simulink model "sbc_uja113x_mode_control_s32k148"  (Simulink 9.0)
settings: Solver=FixedStepDiscrete  StartTime=0.0  StopTime=10.0  FixedStep=0.1  RelTol=1e-3
InitFcn:
  | mbd_s32k_consistency_checks(bdroot(gcs));
undefined symbols (not defined in the file): bit, LQFP
libraries: mbd_s32k1xx_ec_toolbox x12, mbd_sbc_ec_toolbox x7, simulink x1
Description:
  | This model demonstrates how to handle operating modes of SBC.
  | 
  | Validation:
  | - A BLUE led is toggled at each time Watchdog resets
  | - Press SW3 to send SBC in Standby mode (RED led should be on)
  | - Press SW4 to send SBC in Normal mode (GREEN led should be on)
  | 
  | Note:
  | This application flashes the non-volatile memory MTPNV and configures the SBC in non-FNMC mode.
  | While the SBC is in non-FNMC mode, the device starts to pull the reset line.
  | It is recommended to clear the MTPNV memory, after this example.
  | 
  |  Erasing the MTPNV memory:
  |  - Connect J11-1 (CANH) to J13-2 (LIN1 VBAT)
  |  - Connect J11-2 (CANL) to J11-4 (GND)
  |  - Push and hold down the reset button SW5
  |  - Turn off and on  the 12V power supply
  |  - Release the reset button and remove the jumper wires
  | 
  | HW prerequisite:
  | - S32k148EVB
  | - One Power Adapter 12V
settings Model: Creator=nxf35375  LastModifiedBy=nxf35172
settings DataIOCC: ExternalInput=off  InitialState=off  SaveFormat=Dataset  SaveOutput=off  SignalLogging=off  SaveTime=off
settings OptimizationCC: DefaultParameterBehavior=Inlined  PassReuseOutputArgsAs=Individual arguments  LifeSpan=auto
settings DebuggingCC: UnderspecifiedInitializationDetection=Simplified  MergeDetectMultiDrivingBlocksExec=error  InheritedTsInSrcMsg=none  SingleTaskRateTransMsg=error  ParameterTunabilityLossMsg=error  UnconnectedInputMsg=error  UnconnectedOutputMsg=error  UnconnectedLineMsg=error  UnknownTsInhSupMsg=error  SFUnexpectedBacktrackingDiag=error  SFNoUnconditionalDefaultTransitionDiag=error  SFExecutionAtInitializationDiag=warning
settings HardwareCC: ProdLargestAtomicInteger=Long  ProdLargestAtomicFloat=Double  ProdIntDivRoundTo=Zero  ProdEndianess=LittleEndian  ProdHWDeviceType=ARM Compatible->ARM Cortex
settings ModelReferenceCC: PropagateSignalLabelsOutOfModel=on
settings SFSimCC: MATLABDynamicMemAlloc=off
settings RTWCC: SystemTargetFile=mbd_s32k.tlc  MakeCommand=mbd_s32k_make_rtw COPY_MDLREF_INCLUDES=0  TemplateMakefile=mbd_s32k.tmf  Description=Model Based Design Toolbox S32K14x Code Generation Target  GenerateReport=on  IncludeHyperlinkInReport=on  LaunchReport=on  GenerateTraceInfo=on  GenerateTraceReport=on  GenerateTraceReportSl=on  GenerateTraceReportSf=on  GenerateTraceReportEml=on
settings CodeAppCC: ForceParamTrailComments=on  IgnoreCustomStorageClasses=off  OperatorAnnotations=on  SimulinkDataObjDesc=on  SFDataObjDesc=on  InsertBlockDesc=on  StateflowObjectComments=off
settings STFCustomTargetCC: TargetLangStandard=C99 (ISO)  MultiwordLength=256  CombineOutputUpdateFcns=on  ERTCustomFileBanners=on  SupportContinuousTime=off  SupportNonInlinedSFcns=off  RemoveResetFunc=on  MATLABClassNameForMDSCustomization=Simulink.SoftwareTarget.ERTCustomization  GRTInterface=off  SystemTargetFile=mbd_s32k.tlc
settings ERTTargetCC: TargetLangStandard=C99 (ISO)  ParMdlRefBuildCompliant=off  CompOptLevelCompliant=off  ConcurrentExecutionCompliant=off  ModelStepFunctionPrototypeControlCompliant=off  CPPClassGenCompliant=off  UseToolchainInfoCompliant=off  InlinedParameterPlacement=NonHierarchical  ERTSrcFileBannerTemplate=mbd_ert_code_template.cgt  ERTHdrFileBannerTemplate=mbd_ert_code_template.cgt  ERTDataSrcFileTemplate=mbd_ert_code_template.cgt  ERTDataHdrFileTemplate=mbd_ert_code_template.cgt  ERTCustomFileTemplate=example_file_process.tlc
settings ConfigComp: CovMetricSettings=dwe  CovHtmlReporting=off  CovSaveCumulativeToWorkspaceVar=off  CovSaveSingleToWorkspaceVar=off  CovExternalEMLEnable=on

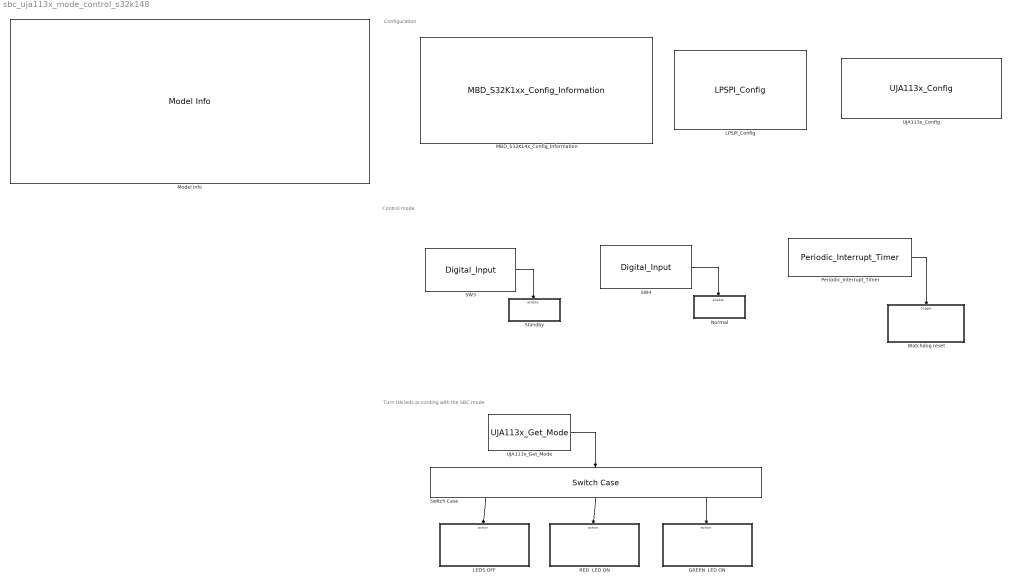
== system sbc_uja113x_mode_control_s32k148 ==
  note: Configuration
  note: Control mode
  note: Turn ON leds according with the SBC mode
  GREEN  LED ON : Subsystem  TreatAsAtomicUnit=on
  LEDS OFF : Subsystem  TreatAsAtomicUnit=on
  "LPSPI_Config " : mbd_s32k1xx_ec_toolbox/Communication Blocks/SPI Blocks/LPSPI_Config   Priority=1  InstanceNumber=1  Role=Master  BaudRate=4000000  ShowAdvanced=on  sin=PTA29: [LPSPI1_SIN | LPSPI Serial Data Input]  sout=PTA27: [LPSPI1_SOUT | LPSPI Serial Data Output]  sck=PTA28: [LPSPI1_SCK | LPSPI Serial Clock I/O]  pcs0=PTA26: [LPSPI1_PCS0 | Peripheral Chip Select 0]  pcs1=None  pcs2=None  pcs3=None  CPHA=1  CPOL=0  BitOrder=MSB first  TransferSize=8  WhichPCS=0  PCSPol=ActiveLow  ContinuousTransfer=on
  MBD_S32K14x_Config_Information : mbd_s32k1xx_ec_toolbox/MBD_S32K1xx_Config_Information  mbdt_ver=0  disp_str=|  config_params=[]  mcu_target_name=S32K148  mcu_target_package=144-LQFP  mcu_target_sram_size=192KB  mcu_system_clock_freq=80  mcu_xtal_freq=External 8  mcu_steptick_timer=LPIT Channel 0  mcu_steptick_prio=15  ds_import_enable=on  target_compiler=GCC  target_memory=FLASH  gcc_target_compile_opts=-mcpu=cortex-m4 -mthumb -mfloat-abi=hard -mfpu=fpv4-sp-d16 -O1 -g -gstrict-dwarf  gcc_target_assemble_opts=-mcpu=cortex-m4 -mthumb -mfloat-abi=hard -mfpu=fpv4-sp-d16 -g  gcc_target_link_opts=-mcpu=cortex-m4 -mthumb -mfloat-abi=hard -mfpu=fpv4-sp-d16  gcc_target_default_lcf=on  gcc_target_user_lcf=S32K148_192_flash.ld  ghs_target_compile_opts=-cpu=cortexm4f -thumb -DARM_MATH_CM4 -fpu=vfpv4_d16 -fsingle -Ogeneral -Wundef -Wimplicit-int -Wshadow -Wtrigraphs --no_commons --gnu_asm -gnu99 -gdwarf-2 -G  ghs_target_assemble_opts=-cpu=cortexm4f -fpu=vfpv4_d16  ghs_target_link_opts=-cpu=cortexm4f -thumb -fpu=vfpv4_d16  ghs_target_default_lcf=off  ghs_target_user_lcf=S32K148_192_flash.ld  iar_target_compile_opts=--cpu=Cortex-M4F --thumb --fpu=VFPv4_sp -Ol -e --debug --dlib_config normal  iar_target_assemble_opts=--cpu Cortex-M4F --thumb --fpu VFPv4_sp  iar_target_link_opts=--no_exceptions --vfe --inline  iar_target_default_lcf=off  iar_target_user_lcf=S32K148_192_flash.icf  pil_download_enable=off  rbl_download_enable=on  rbl_start_delay=5000000  rbl_download_interface=OpenSDA  rbl_restart_request=off  rbl_com_port=Custom  rbl_com_port_custom=COM1  pil_download_rate=57600  pil_opensda_drive=Custom  pil_opensda_drive_custom=D  pil_uart_instance=0  pil_uart_rx=PTA2: [LPUART0_RX | Receive]  pil_uart_tx=PTA3: [LPUART0_TX | Transmit]  FTM_PWM_PcrCheckEnDis=on  FTM_Input_Edge_Inputs_PcrCheckEnDis=off  FTM_Dual_Edge_Inputs_PcrCheckEnDis=off  FTM_Quadrature_Inputs_PcrCheckEnDis=off  FTM_Hall_Sensor_Inputs_PcrCheckEnDis=on  LPTMR_PcrCheckEnDis=off  PIT_PcrCheckEnDis=off  RTC_PcrCheckEnDis=off  FlexCAN_PcrCheckEnDis=off  LIN_PcrCheckEnDis=on  FlexIO_PcrCheckEnDis=off  LPI2C_PcrCheckEnDis=off  LPSPI_PcrCheckEnDis=on  LPUART_PcrCheckEnDis=off  CMP_PcrCheckEnDis=off  GPIO_OutputPcrCheckEnDis=on  GPIO_InputPcrCheckEnDis=on  SBC_PcrCheckEnDis=on  AMMCLIB_PcrCheckEnDis=off  FM_PcrCheckEnDis=off  Profile_PcrCheckEnDis=off  ConfigParams_PcrCheckEnDis=on  ModelRef_PcrCheckEnDis=on  PDB0_PcrCheckEnDis=off  CSEc_PcrCheckEnDis=off  eDMA_PcrCheckEnDis=off  ADC_PcrCheckEnDis=off  WDOG_PcrCheckEnDis=on
      | Target : S32K144-64KB_SRAM
      | Package : 100-pin
      | System clock : 80 MHz
      | XTAL clock : External 8 MHz
      | Compiler : IAR
      | Target Type : FLASH
      | Download Code after build : off
      | Step Tick Interrupt Priority : 15
  Model Info : simulink/Model-Wide Utilities/Model Info  Frame=on  DisplayStringWithTags=|  HorizontalTextAlignment=Left  LeftAlignmentValue=0.02
      | Model Name: %<ModelName>
      | 
      | Description: %<Description>
  Normal : Subsystem  TreatAsAtomicUnit=on
  Periodic_Interrupt_Timer : mbd_s32k1xx_ec_toolbox/Utility Blocks/Periodic_Interrupt_Timer  channel=1  period=3000000  prio=15  startCounter=on
  RED  LED ON : Subsystem  TreatAsAtomicUnit=on
  SW3 : mbd_s32k1xx_ec_toolbox/GPIO Blocks/Digital_Input  gpio_pin=PTC12: [PTC12 | Port C I/O]  pull_resistor=Pulldown  passive_filter=off
  SW4 : mbd_s32k1xx_ec_toolbox/GPIO Blocks/Digital_Input  gpio_pin=PTC13: [PTC13 | Port C I/O]  pull_resistor=Pulldown  passive_filter=off
  Standby : Subsystem  TreatAsAtomicUnit=on
  Switch Case : SwitchCase  CaseConditions={1,4,7}  ShowDefaultCase=off
  UJA113x_Config : mbd_sbc_ec_toolbox/UJA113x/UJA113x_Config  Instance=0  deviceModel=UJA1132HWFD5V0  modeCtrl=NORMAL  LHCtrl=Floating  V2SC=None  VextConfig=OFF  ResetTresh=90  WdogModeCtrl=Window  NominalPer=4096 ms  Lock0=off  Lock1=off  Lock2=off  Lock3=off  Lock4=off  Lock5=off  Lock6=off  FDcontrol=off  FDPartial=off  CANmodeCtrl=Offline  dataRate=50 kbit/s  ID1=0  ID2=0  ID3=0  ID4=0  IDmask1=0  IDmask2=0  IDmask3=0  IDmask4=0  IdFormat=11-bit  PartialNetwData=Don't care  DataLength=0  dataMask0=0  dataMask4=0  dataMask1=0  dataMask5=0  dataMask2=0  dataMask6=0  dataMask3=0  dataMask7=0  V2overv=on  V2underv=on  V1underv=on  CANsilence=on  Lin1WkUp=on  CANfailure=on  Lin2WkUp=on  CANwkUp=on  overtempWrng=on  spiFailure=on  Pins=None  risingEdge=off  fallingEdge=off
  UJA113x_Get_Mode : mbd_sbc_ec_toolbox/UJA113x/UJA113x_Get_Mode
  Watchdog reset : Subsystem
  wires:
  Periodic_Interrupt_Timer/1 -> Watchdog reset/Trigger
  SW3/1 -> Standby/Enable
  SW4/1 -> Normal/Enable
  UJA113x_Get_Mode/1 -> Switch Case/1
  Switch Case/1 -> LEDS OFF/Action
  Switch Case/3 -> GREEN  LED ON/Action
  Switch Case/2 -> RED  LED ON/Action

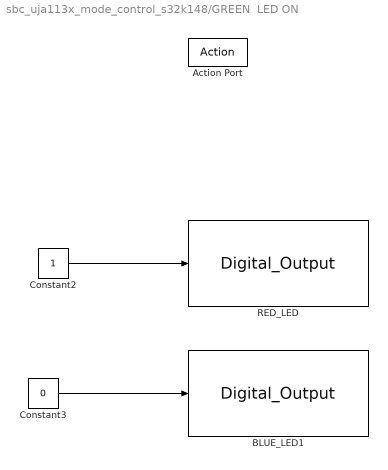
== system sbc_uja113x_mode_control_s32k148/GREEN  LED ON ==
  Action Port : ActionPort  ActionType=case
  BLUE_LED1 : mbd_s32k1xx_ec_toolbox/GPIO Blocks/Digital_Output  Priority=2  gpio_pin=PTE22: [PTE22 | Port E I/O]  init_val=Low  drive_strength=Low
  Constant2 : Constant  OutDataTypeStr=boolean
  Constant3 : Constant  Value=0  OutDataTypeStr=boolean
  RED_LED : mbd_s32k1xx_ec_toolbox/GPIO Blocks/Digital_Output  Priority=2  gpio_pin=PTE21: [PTE21 | Port E I/O]  init_val=Low  drive_strength=Low
  wires:
  Constant2/1 -> RED_LED/1
  Constant3/1 -> BLUE_LED1/1

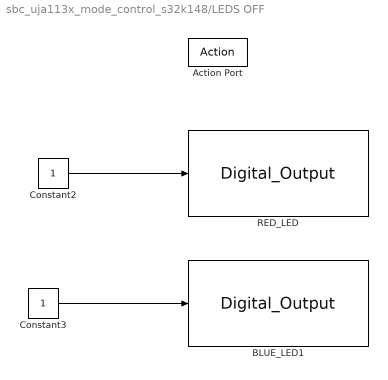
== system sbc_uja113x_mode_control_s32k148/LEDS OFF ==
  Action Port : ActionPort  ActionType=case
  BLUE_LED1 : mbd_s32k1xx_ec_toolbox/GPIO Blocks/Digital_Output  Priority=2  gpio_pin=PTE22: [PTE22 | Port E I/O]  init_val=Low  drive_strength=Low
  Constant2 : Constant  OutDataTypeStr=boolean
  Constant3 : Constant  OutDataTypeStr=boolean
  RED_LED : mbd_s32k1xx_ec_toolbox/GPIO Blocks/Digital_Output  Priority=2  gpio_pin=PTE21: [PTE21 | Port E I/O]  init_val=Low  drive_strength=Low
  wires:
  Constant2/1 -> RED_LED/1
  Constant3/1 -> BLUE_LED1/1

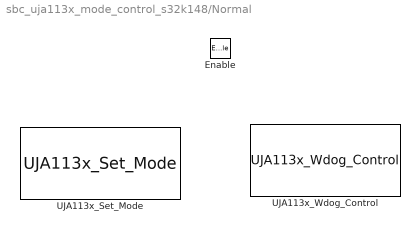
== system sbc_uja113x_mode_control_s32k148/Normal ==
  Enable : EnablePort
  UJA113x_Set_Mode : mbd_sbc_ec_toolbox/UJA113x/UJA113x_Set_Mode  modeCtrl=Normal  status=off
  UJA113x_Wdog_Control : mbd_sbc_ec_toolbox/UJA113x/UJA113x_Wdog_Control  reset=off  mode=on  ModeCtrl=Window  period=off  NominalPer=128 ms

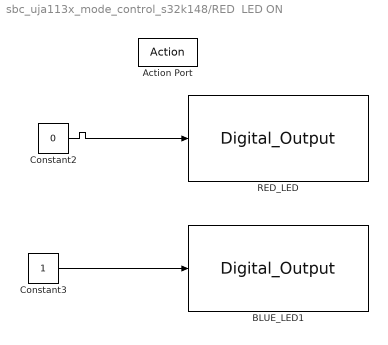
== system sbc_uja113x_mode_control_s32k148/RED  LED ON ==
  Action Port : ActionPort  ActionType=case
  BLUE_LED1 : mbd_s32k1xx_ec_toolbox/GPIO Blocks/Digital_Output  Priority=2  gpio_pin=PTE22: [PTE22 | Port E I/O]  init_val=Low  drive_strength=Low
  Constant2 : Constant  Value=0  OutDataTypeStr=boolean
  Constant3 : Constant  OutDataTypeStr=boolean
  RED_LED : mbd_s32k1xx_ec_toolbox/GPIO Blocks/Digital_Output  Priority=2  gpio_pin=PTE21: [PTE21 | Port E I/O]  init_val=Low  drive_strength=Low
  wires:
  Constant2/1 -> RED_LED/1
  Constant3/1 -> BLUE_LED1/1

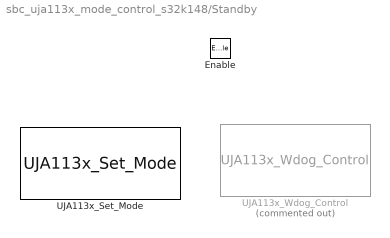
== system sbc_uja113x_mode_control_s32k148/Standby ==
  Enable : EnablePort
  UJA113x_Set_Mode : mbd_sbc_ec_toolbox/UJA113x/UJA113x_Set_Mode  Priority=2  modeCtrl=Standby  status=off
  UJA113x_Wdog_Control : mbd_sbc_ec_toolbox/UJA113x/UJA113x_Wdog_Control  Priority=1  Commented=on  reset=off  mode=on  ModeCtrl=Autonomous  period=off  NominalPer=128 ms

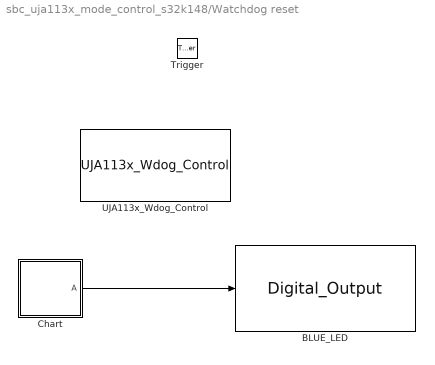
== system sbc_uja113x_mode_control_s32k148/Watchdog reset ==
  Trigger : TriggerPort  TriggerType=function-call  VariantControl=Variant  PortDimensions=1
  BLUE_LED : mbd_s32k1xx_ec_toolbox/GPIO Blocks/Digital_Output  Priority=2  gpio_pin=PTE23: [PTE23 | Port E I/O]  init_val=Low  drive_strength=Low
  Chart : Stateflow chart  TreatAsAtomicUnit=on
  UJA113x_Wdog_Control : mbd_sbc_ec_toolbox/UJA113x/UJA113x_Wdog_Control  Priority=1  reset=on  mode=off  ModeCtrl=Autonomous  period=off  NominalPer=128 ms
  wires:
  Chart/1(" A") -> BLUE_LED/1

== stateflow chart Watchdog reset/Chart ==
  state A
  state A1
  (default) -> A
  A -> A1
  A1 -> A
  data: A output boolean [0..1]
